simulink model "Simulink_Model"  (R2022a)
settings: Solver=VariableStepAuto  StartTime=0.0  StopTime=inf  RelTol=1e-2
values from neighbouring files (symbols this model uses):
  Air_Density = 1.2    [car_and_motor_specifications.mat]
  Angle_of_Inclination = 0    [car_and_motor_specifications.mat]
  Armature_Inductance = 0.001558    [car_and_motor_specifications.mat]
  Armature_Resistence = 0.13    [car_and_motor_specifications.mat]
  Car_Inertia = 72.825    [car_and_motor_specifications.mat]
  Drag_Cofeccient = 0.33    [car_and_motor_specifications.mat]
  Field_Inductance = 13.39    [car_and_motor_specifications.mat]
  Field_Resistence = 84.91    [car_and_motor_specifications.mat]
  Field_Voltage = 300    [car_and_motor_specifications.mat]
  Frontal_Area = 2.2    [car_and_motor_specifications.mat]
  Vehicle_Mass = 860    [car_and_motor_specifications.mat]
  Wheel_Radius = 0.291    [car_and_motor_specifications.mat]
undefined symbols (not defined in the file or in its folder): magnitude
libraries: simulink x2, spsDCMachineLib x1, spsControlledVoltageSourceLib x1, spsDCVoltageSourceLib x1, spspowerguiLib x1
settings Model: Creator=jamesbond  LastModifiedBy=jamesbond
settings DataIOCC: Refine=10

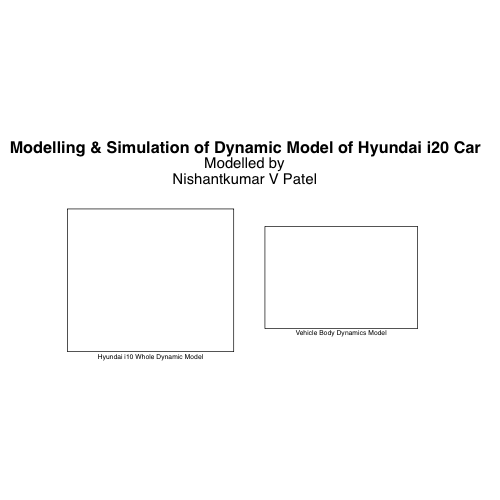
[thumbnail: Simulink's stored preview of the top-level diagram]
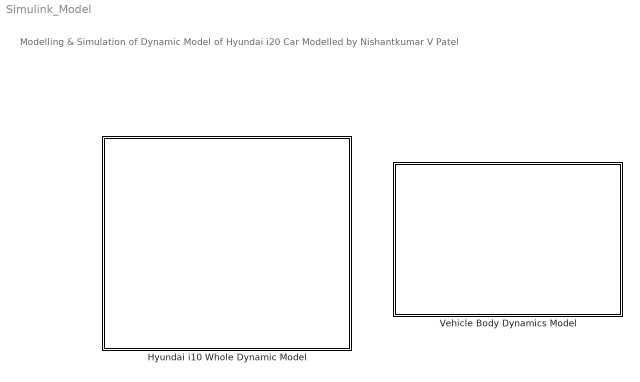
== system Simulink_Model ==
  note: Modelling & Simulation of Dynamic Model of Hyundai i20 Car
      | Modelled by
      | Nishantkumar V Patel
  Hyundai i10 Whole Dynamic Model : Subsystem
  Vehicle Body Dynamics Model : Subsystem

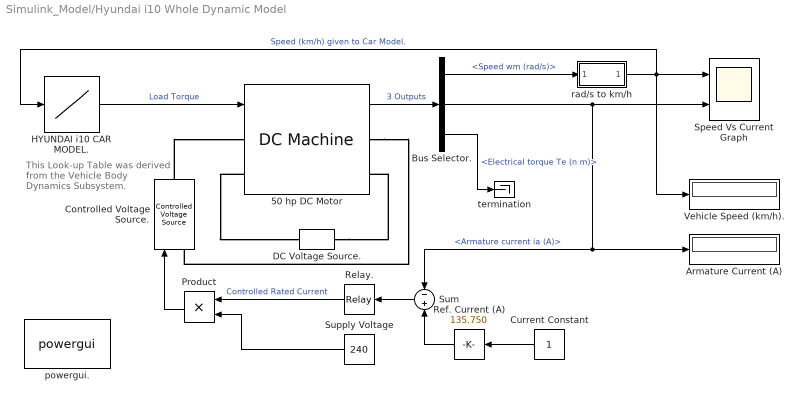
== system Simulink_Model/Hyundai i10 Whole Dynamic Model ==
  note: This Look-up Table was
      |  derived from the Vehicle
      |  Body Dynamics Subsystem.
  50 hp DC Motor : spsDCMachineLib/DC Machine  PresetModel=No  MechanicalLoad=Torque TL  FieldType=Wound  ShowDetailedParameters=on  MeasurementBus=off  RLa=[Armature_Resistence Armature_Inductance]  RLf=[Field_Resistence Field_Inductance]  Laf=Field_Armature_Mutual_Inductance  MachineConstant=Torque constant (N.m/A)  Ke=1.8  Kt=1.8  J=Car_Inertia  Bm=Viscous_Friction_Coefficient  Tf=Friction_Torque  w0=1  Ifinit=3.53315274997056  TsPowergui=0  TsBlock=-1
  Armature Current (A) : Display
  Bus Selector. : BusSelector  OutputSignals=Speed wm (rad/s),Armature current ia (A),Electrical torque Te (n m)
  Controlled Voltage Source. : spsControlledVoltageSourceLib/Controlled Voltage Source  Initialize=on  Source_Type=DC  Amplitude=0  Phase=0  Frequency=0  Measurements=None
  Current Constant : Constant
  DC Voltage Source. : spsDCVoltageSourceLib/DC Voltage Source  Amplitude=Field_Voltage  Measurements=None
  HYUNDAI i10 CAR MODEL. : Lookup_n-D  NumberOfTableDimensions=1  BreakpointsForDimension1=[0 22.61 31.98 39.16 45.22 50.56 55.38 59.82 64 67.83 71.5 75 78.32 81.52 84.6 87.57 90.44 93.22 95.93 101.1]  Table=[0 5 10 15 20 25 30 35 40 45 50 55 60 65 70 75 80 85 90 100]  InternalRulePriority=Speed  RndMeth=Simplest
  Product : Product
  "Ref. Current (A) " : simulink/Math Operations/Slider Gain  gain=135.750  low=0  high=181
  Relay. : Relay  OnSwitchValue=2  OffSwitchValue=-2
  Speed Vs Current Graph : Scope  NumInputPorts=2
  Sum : Sum  Inputs=-+
  Supply Voltage : Constant  Value=240
  Vehicle Speed (km/h). : Display
  powergui. : spspowerguiLib/powergui  Priority=1  SimulationMode=Discrete  SampleTime=50e-6  frequency=60  Iterations=50  frequencyindice=0  Pbase=100e6  ErrMax=1e-4  UnitsV=kV  UnitsW=MW  buscounter=0  FunctionMessages=off  echomessages=off  EnableUseOfTLC=off  CurrentSourceSwitches=off  DisableSnubberDevices=off  DisableRonSwitches=off  DisableVfSwitches=off  DisplayEquations=off  AutomaticDiscreteSolvers=off  SolverType=Tustin/Backward Euler (TBE)  Interpol=off  ExternalGateDelay=off  methode=off  Ts=100  x0status=blocks  SPID=on  SwTol=0  HookPort=off  NonlinearTolerance=1e-4  nMaxIteration=100  ContinueOnMaxIteration=off  RestoreLinks=warning  ResistiveCurrentMeasurement=off  Frange=[0:2:500]  Ylog=off  Xlog=on  ShowGrid=off  save=off  variable=ZData  structure=0  ZoomFFT=off  StartTime=0.0  cycles=1  DisplayStyle=1  fundamental=60  FreqAxis=off  MaxFrequency=1000  frequencyindicesteady=1  RmsSteady=1  display=off
  rad/s to km/h : Subsystem
  termination : Terminator
  wires:
  Current Constant/1 -> "Ref. Current (A) "/1
  50 hp DC Motor/1 -> Bus Selector./1  "3 Outputs"
  Relay./1 -> Product/1  "Controlled Rated Current"
  Supply Voltage/1 -> Product/2
  Bus Selector./3 -> termination/1  "<Electrical torque Te (n m)>"
  rad/s to km/h/1(Out1) -> HYUNDAI i10 CAR MODEL./1, Speed Vs Current Graph/1, Vehicle Speed (km/h)./1  "Speed (km/h) given to Car Model."
  Sum/1 -> Relay./1
  Product/1 -> Controlled Voltage Source./1
  HYUNDAI i10 CAR MODEL./1 -> 50 hp DC Motor/1  "Load Torque"
  "Ref. Current (A) "/1 -> Sum/2
  Bus Selector./1 -> rad/s to km/h/1(<Speed wm (rad/s)>)  "<Speed wm (rad/s)>"
  Bus Selector./2 -> Sum/1, Armature Current (A)/1, Speed Vs Current Graph/2  "<Armature current ia (A)>"
  connections:
  50 hp DC Motor/LConn2 -- DC Voltage Source./RConn1
  50 hp DC Motor/RConn1 -- Controlled Voltage Source./LConn1
  Controlled Voltage Source./RConn1 -- 50 hp DC Motor/LConn1
  DC Voltage Source./LConn1 -- 50 hp DC Motor/RConn2

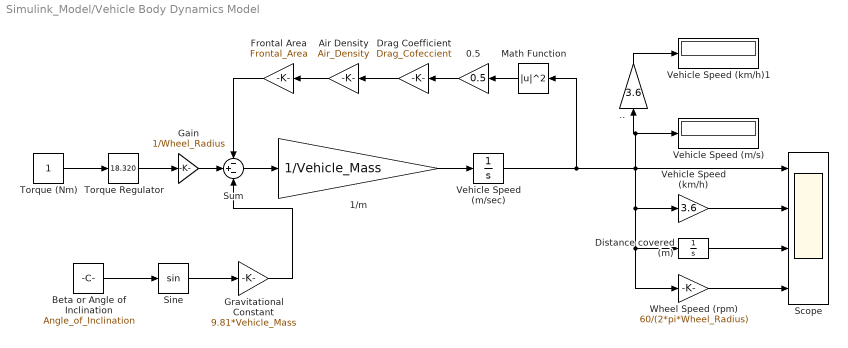
== system Simulink_Model/Vehicle Body Dynamics Model ==
  .. : Gain  Gain=3.6
  0.5 : Gain  Gain=0.5
  1/m : Gain  Gain=1/Vehicle_Mass
  Air Density : Gain  Gain=Air_Density
  Beta or Angle of Inclination : Constant  Value=Angle_of_Inclination
  Distance covered (m) : Integrator
  Drag Coefficient : Gain  Gain=Drag_Cofeccient
  Frontal Area : Gain  Gain=Frontal_Area
  Gain : Gain  Gain=1/Wheel_Radius
  Gravitational Constant : Gain  Gain=9.81*Vehicle_Mass
  Math Function : Math  Operator=magnitude^2
  Scope : Scope  NumInputPorts=4
  Sine : Trigonometry
  Sum : Sum  Inputs=-+-
  Torque (Nm) : Constant
  Torque Regulator : simulink/Math Operations/Slider Gain  gain=18.320  low=0  high=203.55
  Vehicle Speed (km/h) : Gain  Gain=3.6
  Vehicle Speed (km/h)1 : Display
  Vehicle Speed (m/s) : Display
  Vehicle Speed (m/sec) : Integrator
  Wheel Speed (rpm) : Gain  Gain=60/(2*pi*Wheel_Radius)
  wires:
  Torque Regulator/1 -> Gain/1
  Gain/1 -> Sum/2
  Wheel Speed (rpm)/1 -> Scope/4
  Distance covered (m)/1 -> Scope/3
  Beta or Angle of Inclination/1 -> Sine/1
  Vehicle Speed (km/h)/1 -> Scope/2
  ../1 -> Vehicle Speed (km/h)1/1
  Math Function/1 -> 0.5/1
  Gravitational Constant/1 -> Sum/3
  1/m/1 -> Vehicle Speed (m/sec)/1
  Sine/1 -> Gravitational Constant/1
  Torque (Nm)/1 -> Torque Regulator/1
  Frontal Area/1 -> Sum/1
  Sum/1 -> 1/m/1
  0.5/1 -> Drag Coefficient/1
  Drag Coefficient/1 -> Air Density/1
  Vehicle Speed (m/sec)/1 -> ../1, Vehicle Speed (m/s)/1, Scope/1, Vehicle Speed (km/h)/1, Distance covered (m)/1, Wheel Speed (rpm)/1, Math Function/1
  Air Density/1 -> Frontal Area/1

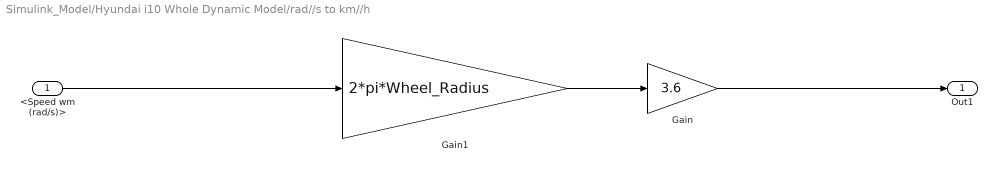
== system Simulink_Model/Hyundai i10 Whole Dynamic Model/rad//s to km//h ==
  <Speed wm (rad/s)> : Inport
  Gain : Gain  Gain=3.6
  Gain1 : Gain  Gain=2*pi*Wheel_Radius
  Out1 : Outport
  wires:
  Gain/1 -> Out1/1
  <Speed wm (rad/s)>/1 -> Gain1/1
  Gain1/1 -> Gain/1
